simulink model "main_sim"  (R2024a)
settings: Solver=VariableStepAuto  StartTime=0.0  StopTime=T  MaxStep=MaxStep  RelTol=RelTol  EnableMultiTasking=on
values from neighbouring files (symbols this model uses):
  a = 0.01    [main.m]
  Emax = 1e6    (= 1000000)    [main.m]
settings Model: Creator=yoash  LastModifiedBy=yoashl
settings SolverCC: AlgebraicLoopSolver=TrustRegion
settings DataIOCC: LimitDataPoints=on  SaveOutput=off  SignalLogging=off  DSMLogging=off  VisualizeSimOutput=off  SaveTime=off  ReturnWorkspaceOutputs=off
settings OptimizationCC: LifeSpan=inf
settings DebuggingCC: UnconnectedInputMsg=warning  UnconnectedOutputMsg=warning  UnconnectedLineMsg=warning  AllowSymbolicDim=off  SFUnexpectedBacktrackingDiag=warning  SFNoUnconditionalDefaultTransitionDiag=warning  SFExecutionAtInitializationDiag=none  ArithmeticOperatorsInVariantConditions=warning
settings ModelReferenceCC: EnableRefExpFcnMdlSchedulingChecks=on  PropagateSignalLabelsOutOfModel=off
settings SFSimCC: SimUseLocalCustomCode=off  CustomCodeUndefinedFunction=UseInterfaceOnly
settings RTWCC: RTWUseLocalCustomCode=off  GPUComputeCapability=3.5  DLArmComputeVersion=19.05
settings CodeAppCC: StateflowObjectComments=on
settings GRTTargetCC: TargetLangStandard=C89/C90 (ANSI)
settings ConfigComp: CovMetricSettings=dw  CovSaveCumulativeToWorkspaceVar=on  CovSaveSingleToWorkspaceVar=on  CovExternalEMLEnable=off

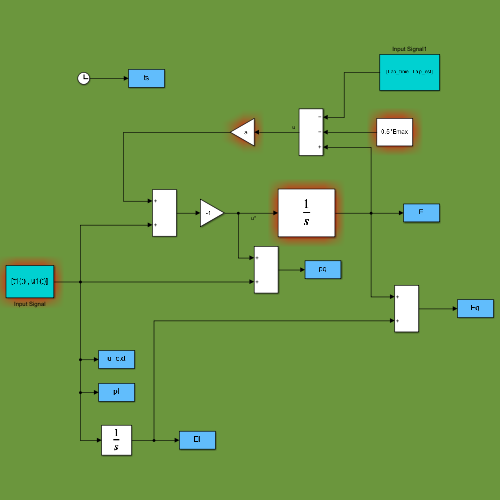
[thumbnail: Simulink's stored preview of the top-level diagram]
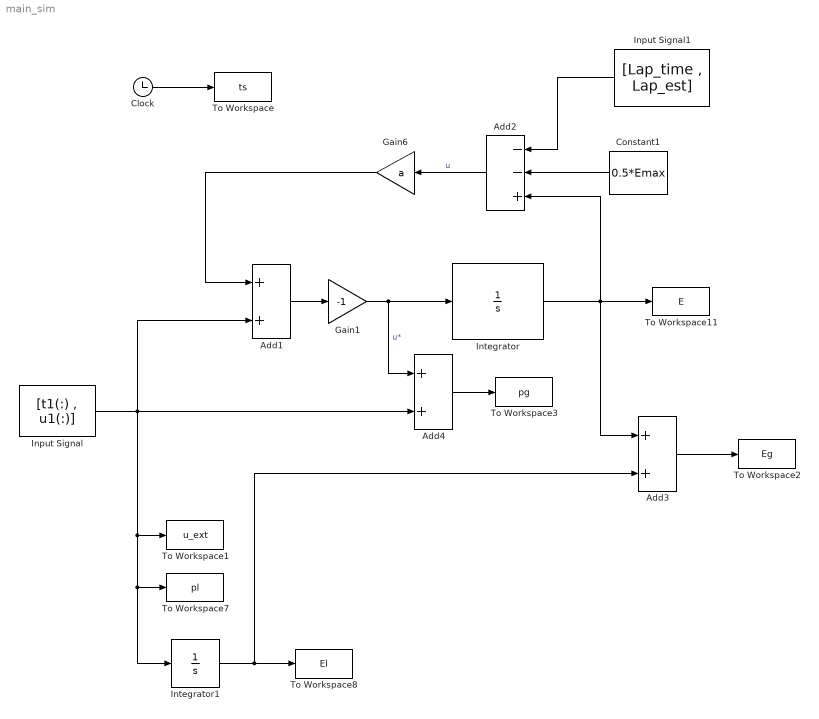
== system main_sim ==
  Add1 : Sum
  Add2 : Sum  Inputs=--+
  Add3 : Sum
  Add4 : Sum
  Clock : Clock
  Constant1 : Constant  Value=0.5*Emax
  Gain1 : Gain  Gain=-1
  Gain6 : Gain  Gain=a
  Input Signal : FromWorkspace  VariableName=[t1(:) , u1(:)]
  Input Signal1 : FromWorkspace  VariableName=[Lap_time , Lap_est]
  Integrator : Integrator  InitialCondition=Emax/2
  Integrator1 : Integrator
  To Workspace : ToWorkspace  VariableName=ts  SampleTime=-1
  To Workspace1 : ToWorkspace  VariableName=u_ext  SampleTime=-1
  To Workspace11 : ToWorkspace  VariableName=E  SampleTime=-1
  To Workspace2 : ToWorkspace  VariableName=Eg  SampleTime=-1
  To Workspace3 : ToWorkspace  VariableName=pg  SampleTime=-1
  To Workspace7 : ToWorkspace  VariableName=pl  SampleTime=-1
  To Workspace8 : ToWorkspace  VariableName=El  SampleTime=-1
  wires:
  Integrator1/1 -> Add3/2, To Workspace8/1
  Integrator/1 -> Add2/3, Add3/1, To Workspace11/1
  Add3/1 -> To Workspace2/1
  Add2/1 -> Gain6/1  "u"
  Gain6/1 -> Add1/1
  Gain1/1 -> Add4/1, Integrator/1  "u*"
  Add1/1 -> Gain1/1
  Clock/1 -> To Workspace/1
  Constant1/1 -> Add2/2
  Add4/1 -> To Workspace3/1
  Input Signal/1 -> Add1/2, Integrator1/1, To Workspace7/1, To Workspace1/1, Add4/2
  Input Signal1/1 -> Add2/1
